simulink model "sampleModel17"  (R2021b)
settings: Solver=VariableStepAuto  StartTime=0.0  StopTime=10.0  RelTol=1e-3
libraries: simulink x12, slpidlib x1
settings Model: Creator=user  LastModifiedBy=user

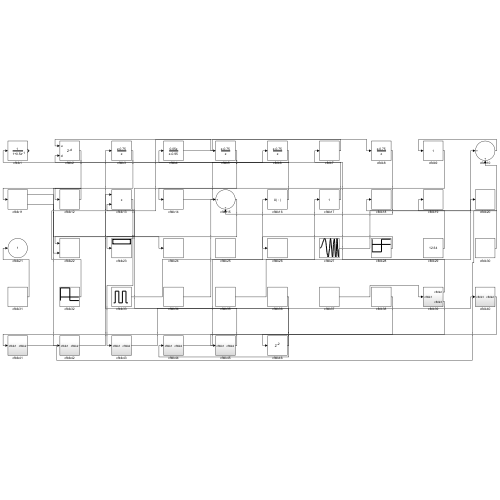
[thumbnail: Simulink's stored preview of the top-level diagram]
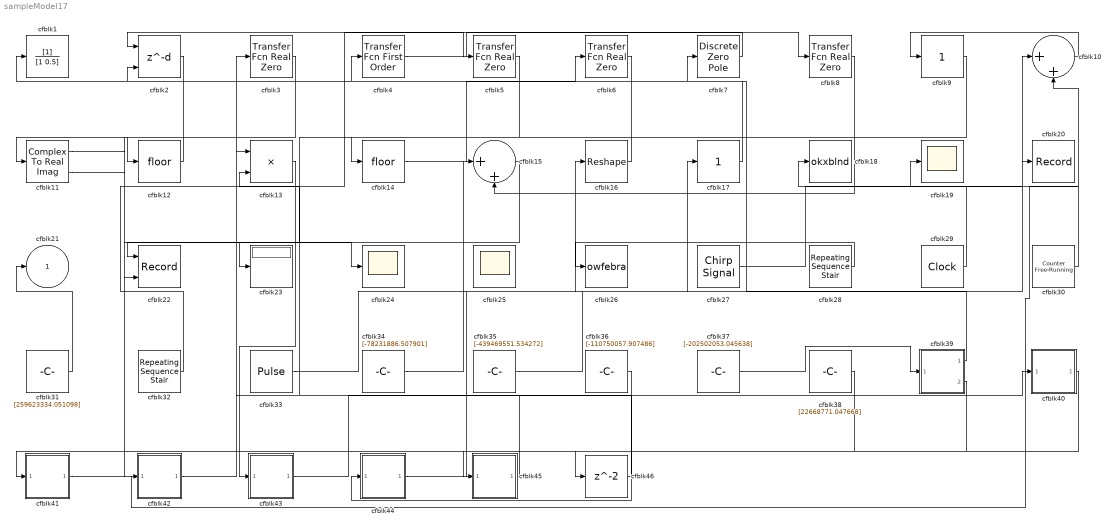
== system sampleModel17 ==
  cfblk1 : DiscreteFilter  SampleTime=1
  cfblk10 : Sum  Inputs=|++
  cfblk11 : ComplexToRealImag
  cfblk12 : Rounding
  cfblk13 : Product
  cfblk14 : Rounding
  cfblk15 : Sum  Inputs=|++
  cfblk16 : Reshape
  cfblk17 : simulink/Math Operations/Slider Gain  gain=1  low=0  high=2
  cfblk18 : ToWorkspace  VariableName=okxblnd  SaveFormat=Timeseries  SampleTime=-1
  cfblk19 : Scope
  cfblk2 : Delay  DelayLengthSource=Input port  SampleTime=1
      settings: InputPortMap=u0,p1
  cfblk20 : Record  FileSettingsInternal="{\"entries\":[{\"content\":{\"excelSettings\":{\"content\":{},\"type\":\"Streamout.ExcelSettings\"}},\"type\":\"Streamout.FileSettingStorage\",\"uuid\":\"17ea2f45-68e3-4bb9-a5b8-5693fa28c361\"}],\"packageUris\":[\"http://schema.mathworks.com/mf0/streamout_blocks/R2020a\"],\"version\":\"1.0\"}"  SignalsInternal="{\"entries\":[{\"content\":{\"signals\":[{\"content\":{\"blockPath\":[\"sampleModel17/cfblk20\"],\"channel\":[],\"dimensions\":[1],\"domain\":\"sampleModel17/cfblk20\",\"lineColor\":\"#ff6929\",\"plots\":[1],\"port\":1,\"sid\":[\"\"],\"signalID\":688,\"signalName\":\"cfblk27\"},\"type\":\"RecordBlkView.Signal\",\"uuid\":\"ff02919d-e522-4283-8259-36fde8ee0fff\"}]},\"type\":\"RecordBlkView.InputSignals\",\"uuid\":\"34ed7dc9-4139-4f60-96ec-8a348516208e\"}],\"packageUris\":[\"http://schema.mathworks.com/mf0/streamout_blocks/R2020a\"],\"version\":\"1.0\"}"  VisualizationBindings="{\"sparklinesplugin\":{\"info\":[{\"bindingParametersList\":[],\"subplotID\":1}]}}"
  cfblk22 : Record  FileSettingsInternal="{\"entries\":[{\"content\":{\"excelSettings\":{\"content\":{},\"type\":\"Streamout.ExcelSettings\"}},\"type\":\"Streamout.FileSettingStorage\",\"uuid\":\"5055ea9d-e812-413b-8fb1-7f1005ad629c\"}],\"packageUris\":[\"http://schema.mathworks.com/mf0/streamout_blocks/R2020a\"],\"version\":\"1.0\"}"  Layout=[1 1]  SignalsInternal="{\"entries\":[{\"content\":{\"signals\":[{\"content\":{\"blockPath\":[\"sampleModel17/cfblk22\"],\"channel\":[],\"dimensions\":[1],\"domain\":\"sampleModel17/cfblk22\",\"lineColor\":\"#a2142f\",\"plots\":[1],\"port\":1,\"sid\":[\"\"],\"signalID\":680,\"signalName\":\"cfblk15\"},\"type\":\"RecordBlkView.Signal\",\"uuid\":\"78bbdca0-42b0-46e0-b451-675e35c684db\"},{\"content\":{\"blockPath\":[\"sampleModel17/cfblk22\"],\"channel\":[],\"dimensions\":[1],\"domain\":\"sampleModel17/cfblk22\",\"lineColor\":\"#139fff\",\"plots\":[1],\"port\":2,\"sid\":[\"\"],\"signalID\":684,\"signalName\":\"cfblk3\"},\"type\":\"RecordBlkView.Signal\",\"uuid\":\"df04af4f-55cf-444e-aa6a-6745dac8366a\"}]},\"type\":\"RecordBlkView.InputSignals\",\"uuid\":\"cdcfe083-e4cf-4232-b9ea-9ed5e2f24395\"}],\"packageUris\":[\"http://schema.mathworks.com/mf0/streamout_blocks/R2020a\"],\"version\":\"1.0\"}"  VisualizationBindings="{\"xyplotplugin\":{\"info\":[{\"series\":[{\"bindingParametersList\":[{\"parameter\":\"X-Axis\",\"signalID\":680,\"signalName\":\"cfblk15\"},{\"parameter\":\"Y-Axis\",\"signalID\":684,\"signalName\":\"cfblk3\"}],\"seriesID\":51880}],\"subplotID\":1}]}}"  CompatibilityTag=XY
  cfblk23 : Display
  cfblk24 : Scope
  cfblk25 : Scope
      settings: Floating=on
  cfblk26 : ToWorkspace  VariableName=owfebra  SaveFormat=Timeseries  SampleTime=-1
  cfblk27 : simulink/Sources/Chirp Signal  f1=[-417794126.870751]  T=[947647653.203563]  f2=[529280908.539559]
  cfblk28 : simulink/Sources/Repeating Sequence Stair  OutValues=[-512632139.581316, 364232122.099020]  tsamp=-1  OutMin=[]  OutMax=[]  OutDataTypeStr=double  OutputDataTypeScalingMode=double  OutDataType=fixdt(0,8)  ConRadixGroup=Best Precision: Vector-wise  OutScaling=2^-12
  cfblk29 : DigitalClock
  cfblk{3,5..6,8} (4 alike) : simulink/Discrete/Transfer Fcn Real Zero  ZeroZ=0.75  ICPrevInput=0.0  DoSatur=off
      settings: SourceProductBaseCode=SL
  cfblk30 : simulink/Sources/Counter Free-Running  NumBits=[9.000000]  tsamp=-1
  cfblk31 : Constant  Value=[259623334.051098]  SampleTime=1
  cfblk32 : simulink/Sources/Repeating Sequence Stair  OutValues=[799596666.540720, -303263195.536271]  tsamp=-1  OutMin=[]  OutMax=[]  OutDataTypeStr=double  OutputDataTypeScalingMode=double  OutDataType=fixdt(0,8)  ConRadixGroup=Best Precision: Vector-wise  OutScaling=2^-12
  cfblk33 : DiscretePulseGenerator  PulseType=Time based  Amplitude=[-27379613.426073]  Period=[67951749.553944]  PulseWidth=5  PhaseDelay=[7.000000]
  cfblk34 : Constant  Value=[-78231886.507901]  SampleTime=1
  cfblk35 : Constant  Value=[-439469551.534272]  SampleTime=1
  cfblk36 : Constant  Value=[-110750057.907486]  SampleTime=1
  cfblk37 : Constant  Value=[-202502053.045638]  SampleTime=1
  cfblk38 : Constant  Value=[22668771.047668]  SampleTime=1
  cfblk39 : Subsystem
  cfblk4 : simulink/Discrete/Transfer Fcn First Order  PoleZ=0.95  ICPrevOutput=0.0  DoSatur=off
  cfblk40 : Subsystem
  cfblk41 : Subsystem
  cfblk42 : Subsystem
  cfblk43 : Subsystem
  cfblk44 : Subsystem
  cfblk45 : Subsystem
  cfblk46 : Delay  SampleTime=1
  cfblk7 : DiscreteZeroPole  Poles=[0 0.5]  Gain=1
  cfblk9 : simulink/Math Operations/Slider Gain  gain=1  low=0  high=2
  cfblk21 : Outport
  wires:
  cfblk35/1 -> cfblk10/1
  cfblk15/1 -> cfblk22/1
  cfblk44/1(cfblk2) -> cfblk16/1
  cfblk36/1 -> cfblk44/1(cfblk1)
  cfblk2/1 -> cfblk12/1
  cfblk29/1 -> cfblk19/1
  cfblk41/1(cfblk2) -> cfblk10/2
  cfblk31/1 -> cfblk21/1
  cfblk4/1 -> cfblk8/1
  cfblk10/1 -> cfblk9/1
  cfblk6/1 -> cfblk4/1
  cfblk30/1 -> cfblk18/1
  cfblk32/1 -> cfblk5/1
  cfblk38/1 -> cfblk41/1(cfblk1)
  cfblk12/1 -> cfblk11/1
  cfblk14/1 -> cfblk6/1
  cfblk9/1 -> cfblk14/1
  cfblk13/1 -> cfblk43/1(cfblk1)
  cfblk33/1 -> cfblk17/1
  cfblk7/1 -> cfblk2/1
  cfblk28/1 -> cfblk26/1
  cfblk42/1(cfblk2) -> cfblk3/1
  cfblk27/1 -> cfblk20/1
  cfblk5/1 -> cfblk23/1
  cfblk17/1 -> cfblk1/1
  cfblk16/1 -> cfblk2/2
  cfblk37/1 -> cfblk39/1(cfblk1)
  cfblk39/1(cfblk2) -> cfblk7/1
  cfblk34/1 -> cfblk15/1
  cfblk43/1(cfblk2) -> cfblk40/1(cfblk1)
  cfblk45/1(cfblk2) -> cfblk13/2
  cfblk3/1 -> cfblk22/2
  cfblk11/1 -> cfblk24/1
  cfblk8/1 -> cfblk15/2
  cfblk11/2 -> cfblk42/1(cfblk1)
  cfblk39/2(cfblk3) -> cfblk45/1(cfblk1)
  cfblk40/1(cfblk2) -> cfblk46/1
  cfblk46/1 -> cfblk13/1

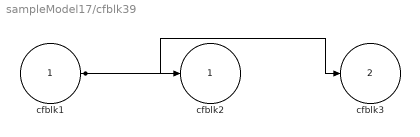
== system sampleModel17/cfblk39 ==
  cfblk1 : Inport
  cfblk2 : Outport
  cfblk3 : Outport  Port=2
  wires:
  cfblk1/1 -> cfblk2/1, cfblk3/1

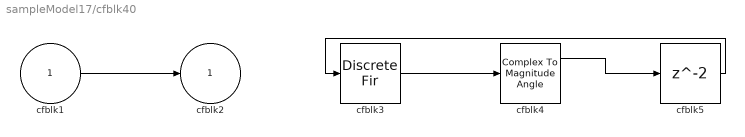
== system sampleModel17/cfblk40 ==
  cfblk1 : Inport
  cfblk3 : DiscreteFir  SampleTime=1
  cfblk4 : ComplexToMagnitudeAngle
  cfblk5 : Delay  SampleTime=1
  cfblk2 : Outport
  wires:
  cfblk1/1 -> cfblk2/1
  cfblk3/1 -> cfblk4/1
  cfblk4/1 -> cfblk5/1
  cfblk5/1 -> cfblk3/1

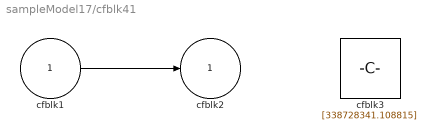
== system sampleModel17/cfblk41 ==
  cfblk1 : Inport
  cfblk3 : Constant  Value=[338728341.108815]  SampleTime=1
  cfblk2 : Outport
  wires:
  cfblk1/1 -> cfblk2/1

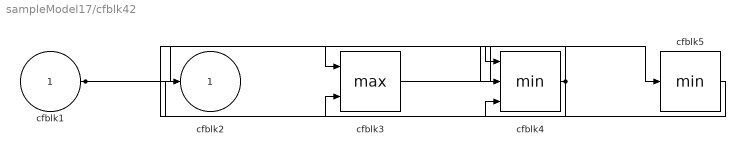
== system sampleModel17/cfblk42 ==
  cfblk1 : Inport
  cfblk3 : MinMax  Function=max  Inputs=2
  cfblk4 : MinMax  Inputs=3
  cfblk5 : MinMax
  cfblk2 : Outport
  wires:
  cfblk3/1 -> cfblk5/1
  cfblk1/1 -> cfblk4/1, cfblk4/2, cfblk4/3
  cfblk5/1 -> cfblk2/1
  cfblk4/1 -> cfblk3/1, cfblk3/2

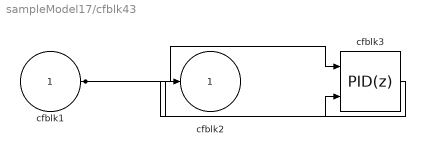
== system sampleModel17/cfblk43 ==
  cfblk1 : Inport
  cfblk3 : slpidlib/PID Controller (2DOF)  Controller=PID  Form=Parallel  TimeDomain=Discrete-time  UseExternalTs=off  SampleTime=1  IntegratorMethod=Forward Euler  FilterMethod=Forward Euler  ControllerParametersSource=internal  P=1  I=1  D=0  UseFilter=on  N=100  b=1  c=1  TunerSelectOption=Transfer Function Based (PID Tuner App)  InitialConditionSource=internal  InitialConditionForIntegrator=0  InitialConditionForFilter=0  DifferentiatorICPrevScaledInput=0  ExternalReset=none  TrackingMode=off  Kt=1  LimitOutput=off  SatLimitsSource=internal  UpperSaturationLimit=inf  LowerSaturationLimit=-inf  LinearizeAsGain=off  AntiWindupMode=none  Kb=1  POutMin=[]  POutMax=[]  IOutMin=[]  IOutMax=[]  DOutMin=[]  DOutMax=[]  NOutMin=[]  NOutMax=[]  bOutMin=[]  bOutMax=[]  cOutMin=[]  cOutMax=[]  SumOutMin=[]  SumOutMax=[]  SaturationOutMin=[]  SaturationOutMax=[]  PParamMin=[]  PParamMax=[]  IParamMin=[]  IParamMax=[]  DParamMin=[]  DParamMax=[]  NParamMin=[]  NParamMax=[]  bParamMin=[]  bParamMax=[]  cParamMin=[]  cParamMax=[]  KbParamMin=[]  KbParamMax=[]  KtParamMin=[]  KtParamMax=[]  KbOutMin=[]  KbOutMax=[]  KtOutMin=[]  KtOutMax=[]  IntegratorOutMin=[]  IntegratorOutMax=[]  FilterOutMin=[]  FilterOutMax=[]  SumI1OutMin=[]  SumI1OutMax=[]  SumI2OutMin=[]  SumI2OutMax=[]  SumI3OutMin=[]  SumI3OutMax=[]  SumI4OutMin=[]  SumI4OutMax=[]  SumDOutMin=[]  SumDOutMax=[]  Sum1OutMin=[]  Sum1OutMax=[]  Sum2OutMin=[]  Sum2OutMax=[]  Sum3OutMin=[]  Sum3OutMax=[]  DifferentiatorOutMin=[]  DifferentiatorOutMax=[]  FilterDiffOutCoefMin=[]  FilterDiffOutCoefMax=[]  ReciprocalOutMin=[]  ReciprocalOutMax=[]  SumDenOutMin=[]  SumDenOutMax=[]  SumNumOutMin=[]  SumNumOutMax=[]  DivideOutMin=[]  DivideOutMax=[]  UdiffTsProdOutMin=[]  UdiffTsProdOutMax=[]  NTsProdOutMin=[]  NTsProdOutMax=[]  UintegralTsProdOutMin=[]  UintegralTsProdOutMax=[]  UngainTsProdOutMin=[]  UngainTsProdOutMax=[]  IntegratorContinuousStateAttributes=''  IntegratorStateMustResolveToSignalObject=off  IntegratorRTWStateStorageClass=Auto  FilterContinuousStateAttributes=''  FilterStateMustResolveToSignalObject=off  FilterRTWStateStorageClass=Auto  ParallelPVariant=InternalParameters  IdealPVariant=Disabled  IVariant=InternalParameters  DVariant=InternalParameters  bVariant=InternalParameters  cVariant=InternalParameters  IntegratorVariant=Discrete  SatVariant=Disabled  AWVariant=Passthrough  PCopyVariant=Disabled  TRVariant=Disabled  FdbkBlocksVariant=Forward  IdealPFdbkVariant=Disabled  SatFdbkVariant=Disabled  DerivativeFilterVariant=ForwardEulerFilter  NVariant=InternalParameters  NCopyVariant=Disabled  FilterICVariant=InternalICsFilter  IntegratorICVariant=InternalICs  ExternalResetVariant=Disabled  TRSumVariant=Passthrough  SumFdbkVariant=Disabled  SumVariant=Sum_PID  TsampFilterVariant=InternalTs  TsampNgainVariant=Passthrough  TsampIntegralVariant=Passthrough  ExternalSaturationOutDataTypeStr=Inherit: Same as second input
      settings: SourceProductBaseCode=SL
  cfblk2 : Outport
  wires:
  cfblk1/1 -> cfblk3/1, cfblk3/2
  cfblk3/1 -> cfblk2/1

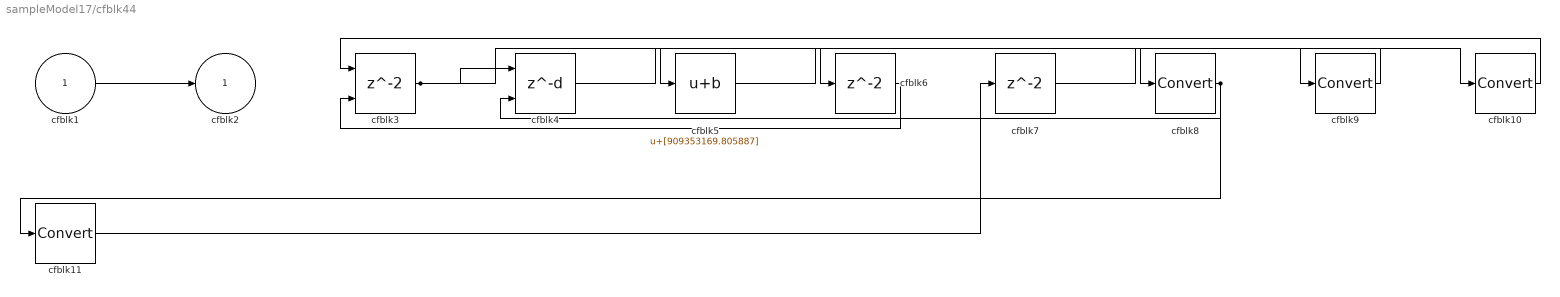
== system sampleModel17/cfblk44 ==
  cfblk1 : Inport
  cfblk{8..11} (4 alike) : DataTypeConversion
  cfblk3 : Delay  ShowEnablePort=on  SampleTime=1
      settings: InputPortMap=u0,e6
  cfblk4 : Delay  DelayLengthSource=Input port  SampleTime=1
      settings: InputPortMap=u0,p1
  cfblk5 : Bias  Bias=[909353169.805887]
  cfblk6 : Delay  SampleTime=1
  cfblk7 : Delay  SampleTime=1
  cfblk2 : Outport
  wires:
  cfblk1/1 -> cfblk2/1
  cfblk3/1 -> cfblk4/1, cfblk9/1
  cfblk5/1 -> cfblk8/1
  cfblk4/1 -> cfblk6/1
  cfblk6/1 -> cfblk3/2
  cfblk8/1 -> cfblk4/2, cfblk11/1
  cfblk9/1 -> cfblk5/1
  cfblk7/1 -> cfblk10/1
  cfblk10/1 -> cfblk3/1
  cfblk11/1 -> cfblk7/1

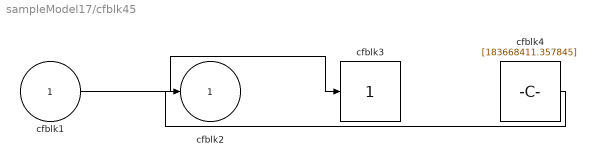
== system sampleModel17/cfblk45 ==
  cfblk1 : Inport
  cfblk3 : simulink/Math Operations/Slider Gain  gain=1  low=0  high=2
  cfblk4 : Constant  Value=[183668411.357845]  SampleTime=1
  cfblk2 : Outport
  wires:
  cfblk1/1 -> cfblk3/1
  cfblk4/1 -> cfblk2/1
